simulink model "EB_12B_with_contracts"  (R2017b)
settings: Solver=ode3  StartTime=0.0  StopTime=0  FixedStep=.01  RelTol=1e-3  EnableMultiTasking=on
model workspace (MAT data in the model file):
  ContractValidatorBlocksMap = containers.Map
  ContractValidatorBlocksMap.serialization.keys = {'EB_12B_with_contracts/EB_12B_EBSpec/validator'}
  ContractValidatorBlocksMap.serialization.values{1}.block = 'EB_12B_with_contracts/EB_12B_EBSpec/validator'
  ContractValidatorBlocksMap.serialization.values{1}.assumePorts = 0
  ContractValidatorBlocksMap.serialization.values{1}.guaranteePorts = 3
  ContractValidatorBlocksMap.serialization.values{1}.modeBlocksPorts = 0
  ContractValidatorBlocksMap.serialization.values{1}.portHandles.Inport = [3286.00024414 3289.00024414 3293.00024414]
  ContractValidatorBlocksMap.serialization.values{1}.portHandles.Outport = 3586.00024414
  ContractValidatorBlocksMap.serialization.values{1}.portHandles.Enable = []
  ContractValidatorBlocksMap.serialization.values{1}.portHandles.Trigger = []
  ContractValidatorBlocksMap.serialization.values{1}.portHandles.State = []
  ContractValidatorBlocksMap.serialization.values{1}.portHandles.LConn = []
  ContractValidatorBlocksMap.serialization.values{1}.portHandles.RConn = []
  ContractValidatorBlocksMap.serialization.values{1}.portHandles.Ifaction = []
  ContractValidatorBlocksMap.serialization.values{1}.portHandles.Reset = []
  ContractValidatorBlocksMap.serialization.values{1}.portConnectivity(1).Type = '1'
  ContractValidatorBlocksMap.serialization.values{1}.portConnectivity(1).Position = [1955 -95]
  ContractValidatorBlocksMap.serialization.values{1}.portConnectivity(1).SrcBlock = 2019.00036621
  ContractValidatorBlocksMap.serialization.values{1}.portConnectivity(1).SrcPort = 0
  ContractValidatorBlocksMap.serialization.values{1}.portConnectivity(1).DstBlock = []
  ContractValidatorBlocksMap.serialization.values{1}.portConnectivity(1).DstPort = []
  ContractValidatorBlocksMap.serialization.values{1}.portConnectivity(2).Type = '2'
  ContractValidatorBlocksMap.serialization.values{1}.portConnectivity(2).Position = [1955 75]
  ContractValidatorBlocksMap.serialization.values{1}.portConnectivity(2).SrcBlock = 2023.00036621
  ContractValidatorBlocksMap.serialization.values{1}.portConnectivity(2).SrcPort = 0
  ContractValidatorBlocksMap.serialization.values{1}.portConnectivity(2).DstBlock = []
  ContractValidatorBlocksMap.serialization.values{1}.portConnectivity(2).DstPort = []
  ContractValidatorBlocksMap.serialization.values{1}.portConnectivity(3).Type = '3'
  ContractValidatorBlocksMap.serialization.values{1}.portConnectivity(3).Position = [1955 245]
  ContractValidatorBlocksMap.serialization.values{1}.portConnectivity(3).SrcBlock = 2031.00036621
  ContractValidatorBlocksMap.serialization.values{1}.portConnectivity(3).SrcPort = 0
  ContractValidatorBlocksMap.serialization.values{1}.portConnectivity(3).DstBlock = []
  ContractValidatorBlocksMap.serialization.values{1}.portConnectivity(3).DstPort = []
  ContractValidatorBlocksMap.serialization.values{1}.portConnectivity(4).Type = '1'
  ContractValidatorBlocksMap.serialization.values{1}.portConnectivity(4).Position = [2090 75]
  ContractValidatorBlocksMap.serialization.values{1}.portConnectivity(4).SrcBlock = []
  ContractValidatorBlocksMap.serialization.values{1}.portConnectivity(4).SrcPort = []
  ContractValidatorBlocksMap.serialization.values{1}.portConnectivity(4).DstBlock = 2226.00024414
  ContractValidatorBlocksMap.serialization.values{1}.portConnectivity(4).DstPort = 0
  ContractValidatorBlocksMap.serialization.uniformity = 0
  ContractValidatorBlocksMap.serialization.keyType = 'char'
  ContractValidatorBlocksMap.serialization.valueType = 'any'
undefined symbols (not defined in the file): contractAfterSimulation, contractBeforeSimulation, ContractBlock, ContractGuaranteeBlock, ContractValidatorBlock, d, I, I0, saveValidatorParameters, up, Wp
libraries: cocosimLibs x2
settings Model: Creator=elliocm  LastModifiedBy=hbourbou
settings DataIOCC: LimitDataPoints=on  SaveFormat=StructureWithTime  SignalLoggingSaveFormat=ModelDataLogs
settings OptimizationCC: LifeSpan=inf
settings DebuggingCC: UnderspecifiedInitializationDetection=Classic  MergeDetectMultiDrivingBlocksExec=none  SolverPrmCheckMsg=warning  MultiTaskDSMMsg=warning  MultiTaskCondExecSysMsg=none  SFUnexpectedBacktrackingDiag=warning  SFNoUnconditionalDefaultTransitionDiag=warning  SFExecutionAtInitializationDiag=none
settings HardwareCC: ProdBitPerPointer=32  ProdBitPerSizeT=32  ProdBitPerPtrDiffT=32  ProdLargestAtomicFloat=None  ProdIntDivRoundTo=Undefined  ProdEndianess=Unspecified  ProdWordSize=32  ProdHWDeviceType=32-bit Generic
settings ModelReferenceCC: PropagateSignalLabelsOutOfModel=off
settings CodeAppCC: StateflowObjectComments=on
settings GRTTargetCC: TargetLangStandard=C89/C90 (ANSI)  GeneratePreprocessorConditionals=Disable all
settings ConfigComp: CovMetricSettings=dw  CovHtmlReporting=on  CovSaveCumulativeToWorkspaceVar=on  CovSaveSingleToWorkspaceVar=on  CovExternalEMLEnable=off  DVMode=PropertyProving  DVTestSuiteOptimization=CombinedObjectives (Nonlinear Extended)

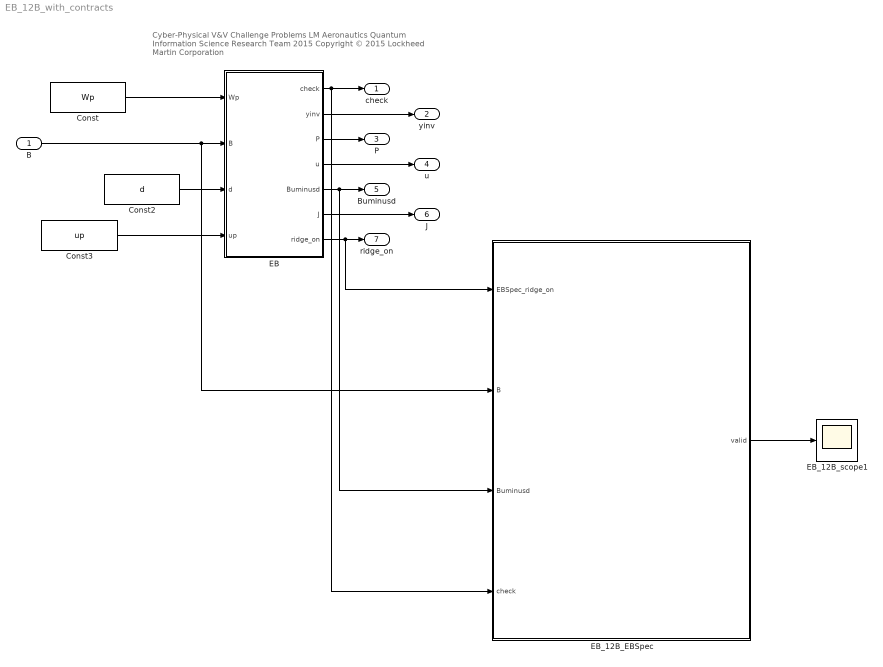
== system EB_12B_with_contracts ==
  note: Cyber-Physical V&V Challenge Problems
      | LM Aeronautics Quantum Information Science Research Team 2015
      | Copyright © 2015 Lockheed Martin Corporation
  B : Inport  OutDataTypeStr=double  PortDimensions=[3 5]
  Const : Constant  Value=Wp
  Const2 : Constant  Value=d
  Const3 : Constant  Value=up
  EB : Subsystem
  EB_12B_EBSpec : Subsystem  mask(ContractBlock){ContractBlockType=ContractBlock}
      mask init:
      | set_param(gcb, 'LinkStatus', 'none');
      mask DialogControl DescTextVar Prompt: Contract block
      mask Display:
      | text(0.5, 0.5, '{\bf\fontsize{20}Contract}', 'hor', 'center', 'texmode','on');
      | blocks = find_system(gcb, 'LookUnderMasks','all', 'SearchDepth',1,'BlockType','Inport');
      | for i = 1 : length(blocks)
      |     blockName = get_param(blocks(i), 'Name');
      |     [path, blockName] = fileparts(char(blockName));
      |     port_label('input', i, blockName);
      | end
      | 
      | blocks = find_system(gcb, 'LookUnderMasks','all', 'SearchDepth',1,'BlockType','Outport');
      | for i = 1 : length(blocks)
      |     blockName = get_param(blocks(i), 'Name');
      |     [path, blockName] = fileparts(char(blockName));
      |     port_label('output', i, blockName);
      | end
  EB_12B_scope1 : Scope
  check : Outport  VectorParamsAs1DForOutWhenUnconnected=off
  yinv : Outport  Port=2  VectorParamsAs1DForOutWhenUnconnected=off
  P : Outport  Port=3  VectorParamsAs1DForOutWhenUnconnected=off
  u : Outport  Port=4  VectorParamsAs1DForOutWhenUnconnected=off
  Buminusd : Outport  Port=5  VectorParamsAs1DForOutWhenUnconnected=off
  J : Outport  Port=6  VectorParamsAs1DForOutWhenUnconnected=off
  ridge_on : Outport  Port=7  VectorParamsAs1DForOutWhenUnconnected=off
  wires:
  Const/1 -> EB/1(Wp)
  B/1 -> EB_12B_EBSpec/2(B), EB/2(B)
  EB/2(yinv) -> yinv/1
  EB/1(check) -> check/1, EB_12B_EBSpec/4(check)
  Const2/1 -> EB/3(d)
  EB/3(P) -> P/1
  EB/4(u) -> u/1
  Const3/1 -> EB/4(up)
  EB/5(Buminusd) -> EB_12B_EBSpec/3(Buminusd), Buminusd/1
  EB/6(J) -> J/1
  EB/7(ridge_on) -> EB_12B_EBSpec/1(EBSpec_ridge_on), ridge_on/1
  EB_12B_EBSpec/1(valid) -> EB_12B_scope1/1

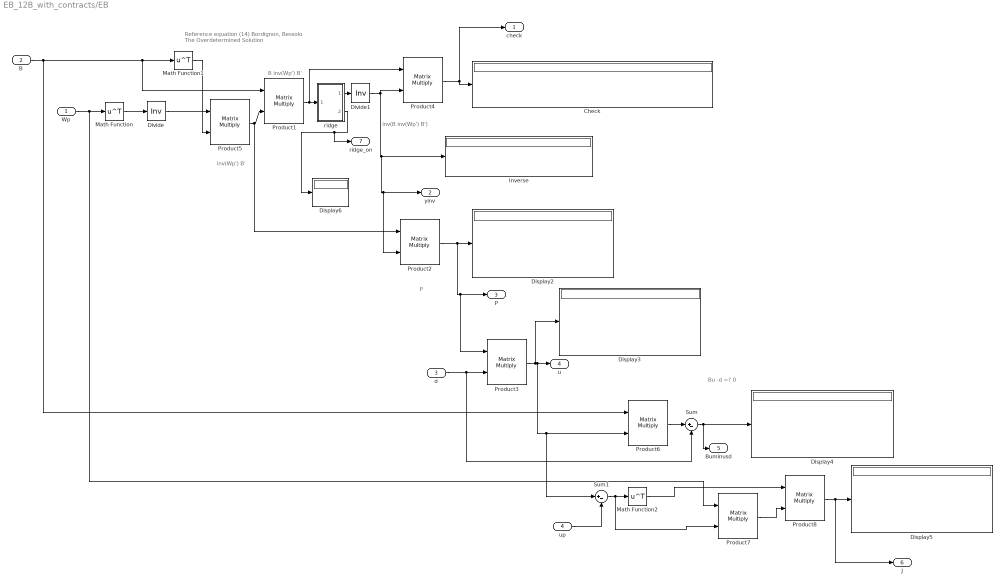
== system EB_12B_with_contracts/EB ==
  note: Reference equation (14) Bordignon, Bessolo
      | The Overdetermined Solution
  note: Bu -d =? 0
  note: P
  note: B inv(Wp') B'
  note: inv(B inv(Wp') B')
  note: inv(Wp') B'
  Wp : Inport
  B : Inport  Port=2
  d : Inport  Port=3
  up : Inport  Port=4
  Check : Display
      settings: Decimation=15
  Display{2..6} (5 alike) : Display
  Divide : Product  Inputs=/  Multiplication=Matrix(*)
  Divide1 : Product  Inputs=/  Multiplication=Matrix(*)
  Inverse : Display
  Math Function : Math  Operator=transpose  SaturateOnIntegerOverflow=on
  Math Function1 : Math  Operator=transpose  SaturateOnIntegerOverflow=on
  Math Function2 : Math  Operator=transpose  SaturateOnIntegerOverflow=on
  Product{1..8} (8 alike) : Product  Multiplication=Matrix(*)
  Sum : Sum  Inputs=|+-
  Sum1 : Sum  Inputs=|+-
  ridge : Subsystem
  check : Outport  VectorParamsAs1DForOutWhenUnconnected=off
  yinv : Outport  Port=2  VectorParamsAs1DForOutWhenUnconnected=off
  P : Outport  Port=3  VectorParamsAs1DForOutWhenUnconnected=off
  u : Outport  Port=4  VectorParamsAs1DForOutWhenUnconnected=off
  Buminusd : Outport  Port=5  VectorParamsAs1DForOutWhenUnconnected=off
  J : Outport  Port=6  VectorParamsAs1DForOutWhenUnconnected=off
  ridge_on : Outport  Port=7  VectorParamsAs1DForOutWhenUnconnected=off
  wires:
  Product1/1 -> Product4/1, ridge/1(In1)
  ridge/1(Out1) -> Divide1/1
  Divide/1 -> Product5/1
  Divide1/1 -> Product2/2, yinv/1, Inverse/1, Product4/2
  Math Function1/1 -> Product5/2
  B/1 -> Product6/1, Product1/1, Math Function1/1
  Math Function/1 -> Divide/1
  Wp/1 -> Product7/1, Math Function/1
  Product5/1 -> Product2/1, Product1/2
  Product4/1 -> check/1, Check/1
  Product2/1 -> Product3/1, P/1, Display2/1
  d/1 -> Sum/2, Product3/2
  Product3/1 -> Display3/1, Sum1/1, Product6/2, u/1
  Product6/1 -> Sum/1
  Sum/1 -> Buminusd/1, Display4/1
  up/1 -> Sum1/2
  Sum1/1 -> Product7/2, Math Function2/1
  Math Function2/1 -> Product8/1
  Product7/1 -> Product8/2
  Product8/1 -> J/1, Display5/1
  ridge/2(ridge_on) -> ridge_on/1, Display6/1

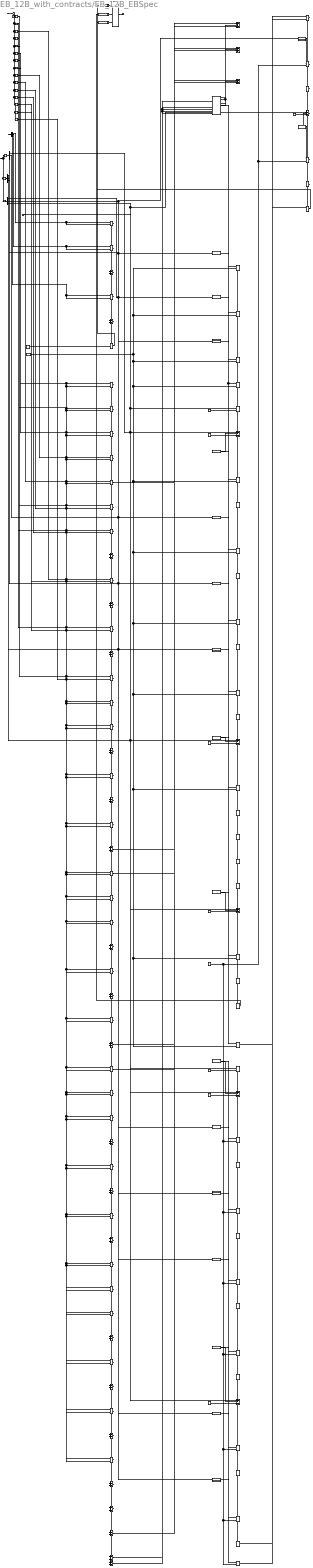
== system EB_12B_with_contracts/EB_12B_EBSpec ==
  EBSpec_ridge_on : Inport  OutDataTypeStr=boolean
  B : Inport  Port=2
  Buminusd : Inport  Port=3
  check : Inport  Port=4
  B_B_T_1_1_operator : Sum  OutDataTypeStr=double
  B_B_T_1_2_operator : Sum  OutDataTypeStr=double
  B_B_T_1_3_operator : Sum  OutDataTypeStr=double
  B_B_T_2_2_operator : Sum  OutDataTypeStr=double
  B_B_T_2_3_operator : Sum  OutDataTypeStr=double
  B_B_T_3_3_operator : Sum  OutDataTypeStr=double
  Buminusd_norm_operator : Sum  OutDataTypeStr=double
  Demux{,1..3} (4 alike) : Demux  Outputs=3
  EB001 : Subsystem  mask(ContractGuaranteeBlock){ContractBlockType=ContractGuaranteeBlock}
      mask init:
      | set_param(gcb, 'LinkStatus', 'none');
      mask DialogControl DescTextVar Prompt: Guarantee block
  EB002 : Subsystem  mask(ContractGuaranteeBlock){ContractBlockType=ContractGuaranteeBlock}
      mask init:
      | set_param(gcb, 'LinkStatus', 'none');
      mask DialogControl DescTextVar Prompt: Guarantee block
  EB004 : Subsystem  mask(ContractGuaranteeBlock){ContractBlockType=ContractGuaranteeBlock}
      mask init:
      | set_param(gcb, 'LinkStatus', 'none');
      mask DialogControl DescTextVar Prompt: Guarantee block
  Selector : Selector  NumberOfDimensions=2  InputPortWidth=3  IndexOptions=Index vector (dialog),Index vector (dialog)  Indices=1,1  OutputSizes=1,1
  Selector1 : Selector  NumberOfDimensions=2  InputPortWidth=3  IndexOptions=Index vector (dialog),Index vector (dialog)  Indices=1,2  OutputSizes=1,1
  Selector10 : Selector  NumberOfDimensions=2  InputPortWidth=3  IndexOptions=Index vector (dialog),Index vector (dialog)  Indices=3,1  OutputSizes=1,1
  Selector11 : Selector  NumberOfDimensions=2  InputPortWidth=3  IndexOptions=Index vector (dialog),Index vector (dialog)  Indices=3,2  OutputSizes=1,1
  Selector12 : Selector  NumberOfDimensions=2  InputPortWidth=3  IndexOptions=Index vector (dialog),Index vector (dialog)  Indices=3,3  OutputSizes=1,1
  Selector13 : Selector  NumberOfDimensions=2  InputPortWidth=3  IndexOptions=Index vector (dialog),Index vector (dialog)  Indices=3,4  OutputSizes=1,1
  Selector14 : Selector  NumberOfDimensions=2  InputPortWidth=3  IndexOptions=Index vector (dialog),Index vector (dialog)  Indices=3,5  OutputSizes=1,1
  Selector15 : Selector  NumberOfDimensions=2  InputPortWidth=3  IndexOptions=Index vector (dialog),Select all  Indices=1,1  OutputSizes=1,1
  Selector16 : Selector  NumberOfDimensions=2  InputPortWidth=3  IndexOptions=Index vector (dialog),Select all  Indices=2,1  OutputSizes=1,1
  Selector17 : Selector  NumberOfDimensions=2  InputPortWidth=3  IndexOptions=Index vector (dialog),Select all  Indices=3,1  OutputSizes=1,1
  Selector2 : Selector  NumberOfDimensions=2  InputPortWidth=3  IndexOptions=Index vector (dialog),Index vector (dialog)  Indices=1,3  OutputSizes=1,1
  Selector3 : Selector  NumberOfDimensions=2  InputPortWidth=3  IndexOptions=Index vector (dialog),Index vector (dialog)  Indices=1,4  OutputSizes=1,1
  Selector4 : Selector  NumberOfDimensions=2  InputPortWidth=3  IndexOptions=Index vector (dialog),Index vector (dialog)  Indices=1,5  OutputSizes=1,1
  Selector5 : Selector  NumberOfDimensions=2  InputPortWidth=3  IndexOptions=Index vector (dialog),Index vector (dialog)  Indices=2,1  OutputSizes=1,1
  Selector6 : Selector  NumberOfDimensions=2  InputPortWidth=3  IndexOptions=Index vector (dialog),Index vector (dialog)  Indices=2,2  OutputSizes=1,1
  Selector7 : Selector  NumberOfDimensions=2  InputPortWidth=3  IndexOptions=Index vector (dialog),Index vector (dialog)  Indices=2,3  OutputSizes=1,1
  Selector8 : Selector  NumberOfDimensions=2  InputPortWidth=3  IndexOptions=Index vector (dialog),Index vector (dialog)  Indices=2,4  OutputSizes=1,1
  Selector9 : Selector  NumberOfDimensions=2  InputPortWidth=3  IndexOptions=Index vector (dialog),Index vector (dialog)  Indices=2,5  OutputSizes=1,1
  abs_call : Subsystem
  abs_call1 : Subsystem
  abs_call11 : Subsystem
  abs_call111 : Subsystem
  abs_call1111 : Subsystem
  abs_call11111 : Subsystem
  abs_call111111 : Subsystem
  abs_call1111111 : Subsystem
  abs_call11111111 : Subsystem
  abs_call111111111 : Subsystem
  abs_call1111111111 : Subsystem
  abs_call11111111111 : Subsystem
  abs_call111111111111 : Subsystem
  abs_call1111111111111 : Subsystem
  abs_call11111111111111 : Subsystem
  abs_call111111111111111 : Subsystem
  abs_call1111111111111111 : Subsystem
  abs_call11111111111111111 : Subsystem
  det_3x3_call : Subsystem
  spec446_operator : cocosimLibs/Implies  SystemSampleTime=-1  Latency=0  AutoFrameSizeCalculation=off
  spec529_operator : cocosimLibs/Implies  SystemSampleTime=-1  Latency=0  AutoFrameSizeCalculation=off
  spec534_operator : RelationalOperator  Operator=<  OutDataTypeStr=boolean  RndMeth=Simplest
  spec534_rhs_2 : Constant  Value=0.0001  OutDataTypeStr=double
  validator : M-S-Function  LoadFcn=saveValidatorParameters(gcb);  InitFcn=contractBeforeSimulation();  StopFcn=contractAfterSimulation();  FunctionName=contract  mask(ContractValidatorBlock){assumePorts=0, guaranteePorts=3, modePorts=0, ContractBlockType=ContractValidatorBlock, createInportsCheckbox=off}
      mask prompts: assumePorts "Assume ports     :"; guaranteePorts "Guarantee ports :"; modePorts "Mode ports        :"; createInportsCheckbox "Create inports and connect them automatically"
      mask init:
      | set_param(gcb,'LinkStatus','none');
      | contract_callback('inputs_callback',gcb);
      mask DialogControl DescTextVar Prompt: The validator block implements the following logic: <br> <br> <b>Sofar</b>(assume<sub>1</sub> <b>&#8743;</b> assume<sub>2</sub> <b>&#8743;</b> ... assume<sub>k</sub>) <b>&rarr;</b> (guarantee<sub>1</sub> <b>&#8743;</b> guarantee<sub>2</sub> <b>&#8743;</b> ... guarantee<sub>m</sub> <b>&#8743;</b>  mode<sub>1</sub> <b>&#8743;</b> mode<sub>2</sub> <b>&#8743;</b> ... <b>&#8743;</b> mode<sub>n</sub> )<br> where mode<sub>i</sub> = require<sub>i</sub> <b>&rarr;</b> ensure<sub>i</sub>
      mask Display:
      | color('black');
      | port_label('input',1,'guarantee');
      | port_label('input',2,'guarantee');
      | port_label('input',3,'guarantee');
      | port_label('output',1,'valid');
  xxEBSpec_100_operator : Sum  OutDataTypeStr=double
  xxEBSpec_101_operator : Sum  OutDataTypeStr=double
  xxEBSpec_102_operator : Sum  OutDataTypeStr=double
  xxEBSpec_103_operator : Product  OutDataTypeStr=double
  xxEBSpec_104_operator : Product  OutDataTypeStr=double
  xxEBSpec_105_operator : Product  OutDataTypeStr=double
  xxEBSpec_106_operator : Product  OutDataTypeStr=double
  xxEBSpec_107_operator : Product  OutDataTypeStr=double
  xxEBSpec_108_operator : Sum  OutDataTypeStr=double
  xxEBSpec_109_operator : Sum  OutDataTypeStr=double
  xxEBSpec_10_operator : Sum  Inputs=+-  OutDataTypeStr=double
  xxEBSpec_10_rhs_2 : Constant  Value=1.0  OutDataTypeStr=double
  xxEBSpec_110_operator : Sum  OutDataTypeStr=double
  xxEBSpec_111_operator : Product  OutDataTypeStr=double
  xxEBSpec_112_operator : Product  OutDataTypeStr=double
  xxEBSpec_113_operator : Product  OutDataTypeStr=double
  xxEBSpec_114_operator : Product  OutDataTypeStr=double
  xxEBSpec_115_operator : Product  OutDataTypeStr=double
  xxEBSpec_116_operator : Sum  OutDataTypeStr=double
  xxEBSpec_117_operator : Sum  OutDataTypeStr=double
  xxEBSpec_118_operator : Sum  OutDataTypeStr=double
  xxEBSpec_12_operator : RelationalOperator  Operator=<  OutDataTypeStr=boolean  RndMeth=Simplest
  xxEBSpec_14_operator : RelationalOperator  Operator=<  OutDataTypeStr=boolean  RndMeth=Simplest
  xxEBSpec_16_operator : RelationalOperator  Operator=<  OutDataTypeStr=boolean  RndMeth=Simplest
  xxEBSpec_18_operator : RelationalOperator  Operator=<  OutDataTypeStr=boolean  RndMeth=Simplest
  xxEBSpec_19_operator : Sum  Inputs=+-  OutDataTypeStr=double
  xxEBSpec_19_rhs_2 : Constant  Value=1.0  OutDataTypeStr=double
  xxEBSpec_1_operator : Sum  Inputs=+-  OutDataTypeStr=double
  xxEBSpec_1_rhs_2 : Constant  Value=1.0  OutDataTypeStr=double
  xxEBSpec_21_operator : RelationalOperator  Operator=<  OutDataTypeStr=boolean  RndMeth=Simplest
  xxEBSpec_22_operator : RelationalOperator  Operator===  OutDataTypeStr=boolean  RndMeth=Simplest
  xxEBSpec_22_rhs_2 : Constant  Value=true  OutDataTypeStr=boolean
  xxEBSpec_23_operator : Logic  AllPortsSameDT=off  OutDataTypeStr=boolean
  xxEBSpec_24_operator : Logic  AllPortsSameDT=off  OutDataTypeStr=boolean
  xxEBSpec_25_operator : Logic  AllPortsSameDT=off  OutDataTypeStr=boolean
  xxEBSpec_26_operator : Logic  AllPortsSameDT=off  OutDataTypeStr=boolean
  xxEBSpec_27_operator : Logic  AllPortsSameDT=off  OutDataTypeStr=boolean
  xxEBSpec_28_operator : Logic  AllPortsSameDT=off  OutDataTypeStr=boolean
  xxEBSpec_29_operator : Logic  AllPortsSameDT=off  OutDataTypeStr=boolean
  xxEBSpec_30_operator : Logic  AllPortsSameDT=off  OutDataTypeStr=boolean
  xxEBSpec_31_operator : Logic  AllPortsSameDT=off  OutDataTypeStr=boolean
  xxEBSpec_32_operator : RelationalOperator  Operator=<=  OutDataTypeStr=boolean  RndMeth=Simplest
  xxEBSpec_33_operator : Sum  Inputs=+-  OutDataTypeStr=double
  xxEBSpec_33_rhs_2 : Constant  Value=1.0  OutDataTypeStr=double
  xxEBSpec_35_operator : RelationalOperator  Operator=<  OutDataTypeStr=boolean  RndMeth=Simplest
  xxEBSpec_37_operator : RelationalOperator  Operator=<  OutDataTypeStr=boolean  RndMeth=Simplest
  xxEBSpec_39_operator : RelationalOperator  Operator=<  OutDataTypeStr=boolean  RndMeth=Simplest
  xxEBSpec_3_operator : RelationalOperator  Operator=<  OutDataTypeStr=boolean  RndMeth=Simplest
  xxEBSpec_41_operator : RelationalOperator  Operator=<  OutDataTypeStr=boolean  RndMeth=Simplest
  xxEBSpec_42_operator : Sum  Inputs=+-  OutDataTypeStr=double
  xxEBSpec_42_rhs_2 : Constant  Value=1.0  OutDataTypeStr=double
  xxEBSpec_44_operator : RelationalOperator  Operator=<  OutDataTypeStr=boolean  RndMeth=Simplest
  xxEBSpec_46_operator : RelationalOperator  Operator=<  OutDataTypeStr=boolean  RndMeth=Simplest
  xxEBSpec_48_operator : RelationalOperator  Operator=<  OutDataTypeStr=boolean  RndMeth=Simplest
  xxEBSpec_50_operator : RelationalOperator  Operator=<  OutDataTypeStr=boolean  RndMeth=Simplest
  xxEBSpec_51_operator : Sum  Inputs=+-  OutDataTypeStr=double
  xxEBSpec_51_rhs_2 : Constant  Value=1.0  OutDataTypeStr=double
  xxEBSpec_53_operator : RelationalOperator  Operator=<  OutDataTypeStr=boolean  RndMeth=Simplest
  xxEBSpec_54_operator : RelationalOperator  Operator===  OutDataTypeStr=boolean  RndMeth=Simplest
  xxEBSpec_54_rhs_2 : Constant  Value=true  OutDataTypeStr=boolean
  xxEBSpec_55_operator : Logic  AllPortsSameDT=off  OutDataTypeStr=boolean
  xxEBSpec_56_operator : Logic  AllPortsSameDT=off  OutDataTypeStr=boolean
  xxEBSpec_57_operator : Logic  AllPortsSameDT=off  OutDataTypeStr=boolean
  xxEBSpec_58_operator : Logic  AllPortsSameDT=off  OutDataTypeStr=boolean
  xxEBSpec_59_operator : Logic  AllPortsSameDT=off  OutDataTypeStr=boolean
  xxEBSpec_5_operator : RelationalOperator  Operator=<  OutDataTypeStr=boolean  RndMeth=Simplest
  xxEBSpec_60_operator : Logic  AllPortsSameDT=off  OutDataTypeStr=boolean
  xxEBSpec_61_operator : Logic  AllPortsSameDT=off  OutDataTypeStr=boolean
  xxEBSpec_62_operator : Logic  AllPortsSameDT=off  OutDataTypeStr=boolean
  xxEBSpec_63_operator : Logic  AllPortsSameDT=off  OutDataTypeStr=boolean
  xxEBSpec_64_operator : RelationalOperator  Operator=<=  OutDataTypeStr=boolean  RndMeth=Simplest
  xxEBSpec_65_operator : Product  OutDataTypeStr=double
  xxEBSpec_66_operator : Product  OutDataTypeStr=double
  xxEBSpec_67_operator : Product  OutDataTypeStr=double
  xxEBSpec_68_operator : Sum  OutDataTypeStr=double
  xxEBSpec_69_rhs : Constant  Value=0.000000000001  OutDataTypeStr=double
  xxEBSpec_70_rhs : Constant  Value=0.000001  OutDataTypeStr=double
  xxEBSpec_71_operator : Product  OutDataTypeStr=double
  xxEBSpec_72_operator : Product  OutDataTypeStr=double
  xxEBSpec_73_operator : Product  OutDataTypeStr=double
  xxEBSpec_74_operator : Product  OutDataTypeStr=double
  xxEBSpec_75_operator : Product  OutDataTypeStr=double
  xxEBSpec_76_operator : Sum  OutDataTypeStr=double
  xxEBSpec_77_operator : Sum  OutDataTypeStr=double
  xxEBSpec_78_operator : Sum  OutDataTypeStr=double
  xxEBSpec_79_operator : Product  OutDataTypeStr=double
  xxEBSpec_7_operator : RelationalOperator  Operator=<  OutDataTypeStr=boolean  RndMeth=Simplest
  xxEBSpec_80_operator : Product  OutDataTypeStr=double
  xxEBSpec_81_operator : Product  OutDataTypeStr=double
  xxEBSpec_82_operator : Product  OutDataTypeStr=double
  xxEBSpec_83_operator : Product  OutDataTypeStr=double
  xxEBSpec_84_operator : Sum  OutDataTypeStr=double
  xxEBSpec_85_operator : Sum  OutDataTypeStr=double
  xxEBSpec_86_operator : Sum  OutDataTypeStr=double
  xxEBSpec_87_operator : Product  OutDataTypeStr=double
  xxEBSpec_88_operator : Product  OutDataTypeStr=double
  xxEBSpec_89_operator : Product  OutDataTypeStr=double
  xxEBSpec_90_operator : Product  OutDataTypeStr=double
  xxEBSpec_91_operator : Product  OutDataTypeStr=double
  xxEBSpec_92_operator : Sum  OutDataTypeStr=double
  xxEBSpec_93_operator : Sum  OutDataTypeStr=double
  xxEBSpec_94_operator : Sum  OutDataTypeStr=double
  xxEBSpec_95_operator : Product  OutDataTypeStr=double
  xxEBSpec_96_operator : Product  OutDataTypeStr=double
  xxEBSpec_97_operator : Product  OutDataTypeStr=double
  xxEBSpec_98_operator : Product  OutDataTypeStr=double
  xxEBSpec_99_operator : Product  OutDataTypeStr=double
  xxEBSpec_9_operator : RelationalOperator  Operator=<  OutDataTypeStr=boolean  RndMeth=Simplest
  valid : Outport
  wires:
  validator/1 -> valid/1
  abs_call/1(abs_y) -> xxEBSpec_9_operator/1
  xxEBSpec_88_operator/1 -> xxEBSpec_94_operator/2
  xxEBSpec_93_operator/1 -> xxEBSpec_94_operator/1
  xxEBSpec_89_operator/1 -> xxEBSpec_93_operator/2
  xxEBSpec_92_operator/1 -> xxEBSpec_93_operator/1
  xxEBSpec_90_operator/1 -> xxEBSpec_92_operator/2
  xxEBSpec_91_operator/1 -> xxEBSpec_92_operator/1
  xxEBSpec_80_operator/1 -> xxEBSpec_86_operator/2
  xxEBSpec_85_operator/1 -> xxEBSpec_86_operator/1
  xxEBSpec_81_operator/1 -> xxEBSpec_85_operator/2
  xxEBSpec_84_operator/1 -> xxEBSpec_85_operator/1
  xxEBSpec_82_operator/1 -> xxEBSpec_84_operator/2
  xxEBSpec_83_operator/1 -> xxEBSpec_84_operator/1
  abs_call1/1(abs_y) -> xxEBSpec_7_operator/1
  xxEBSpec_72_operator/1 -> xxEBSpec_78_operator/2
  xxEBSpec_77_operator/1 -> xxEBSpec_78_operator/1
  xxEBSpec_73_operator/1 -> xxEBSpec_77_operator/2
  xxEBSpec_76_operator/1 -> xxEBSpec_77_operator/1
  xxEBSpec_74_operator/1 -> xxEBSpec_76_operator/2
  xxEBSpec_75_operator/1 -> xxEBSpec_76_operator/1
  xxEBSpec_66_operator/1 -> xxEBSpec_68_operator/2
  xxEBSpec_67_operator/1 -> xxEBSpec_68_operator/1
  xxEBSpec_35_operator/1 -> xxEBSpec_63_operator/2
  xxEBSpec_62_operator/1 -> xxEBSpec_63_operator/1
  xxEBSpec_37_operator/1 -> xxEBSpec_62_operator/2
  xxEBSpec_61_operator/1 -> xxEBSpec_62_operator/1
  xxEBSpec_39_operator/1 -> xxEBSpec_61_operator/2
  xxEBSpec_60_operator/1 -> xxEBSpec_61_operator/1
  xxEBSpec_41_operator/1 -> xxEBSpec_60_operator/2
  xxEBSpec_59_operator/1 -> xxEBSpec_60_operator/1
  abs_call11/1(abs_y) -> xxEBSpec_5_operator/1
  xxEBSpec_44_operator/1 -> xxEBSpec_59_operator/2
  xxEBSpec_58_operator/1 -> xxEBSpec_59_operator/1
  xxEBSpec_46_operator/1 -> xxEBSpec_58_operator/2
  xxEBSpec_57_operator/1 -> xxEBSpec_58_operator/1
  xxEBSpec_48_operator/1 -> xxEBSpec_57_operator/2
  xxEBSpec_56_operator/1 -> xxEBSpec_57_operator/1
  xxEBSpec_50_operator/1 -> xxEBSpec_56_operator/2
  xxEBSpec_55_operator/1 -> xxEBSpec_56_operator/1
  xxEBSpec_53_operator/1 -> xxEBSpec_55_operator/2
  xxEBSpec_54_operator/1 -> xxEBSpec_55_operator/1
  xxEBSpec_54_rhs_2/1 -> xxEBSpec_54_operator/2
  abs_call111111111/1(abs_y) -> xxEBSpec_53_operator/1
  xxEBSpec_51_rhs_2/1 -> xxEBSpec_51_operator/2
  abs_call1111111111/1(abs_y) -> xxEBSpec_50_operator/1
  abs_call11111111111/1(abs_y) -> xxEBSpec_48_operator/1
  abs_call111111111111/1(abs_y) -> xxEBSpec_46_operator/1
  abs_call1111111111111/1(abs_y) -> xxEBSpec_44_operator/1
  xxEBSpec_42_rhs_2/1 -> xxEBSpec_42_operator/2
  abs_call11111111111111/1(abs_y) -> xxEBSpec_41_operator/1
  abs_call11111111/1(abs_y) -> xxEBSpec_3_operator/1
  abs_call111111111111111/1(abs_y) -> xxEBSpec_39_operator/1
  abs_call1111111111111111/1(abs_y) -> xxEBSpec_37_operator/1
  abs_call11111111111111111/1(abs_y) -> xxEBSpec_35_operator/1
  xxEBSpec_33_rhs_2/1 -> xxEBSpec_33_operator/2
  xxEBSpec_3_operator/1 -> xxEBSpec_31_operator/2
  xxEBSpec_30_operator/1 -> xxEBSpec_31_operator/1
  xxEBSpec_5_operator/1 -> xxEBSpec_30_operator/2
  xxEBSpec_29_operator/1 -> xxEBSpec_30_operator/1
  xxEBSpec_7_operator/1 -> xxEBSpec_29_operator/2
  xxEBSpec_28_operator/1 -> xxEBSpec_29_operator/1
  xxEBSpec_9_operator/1 -> xxEBSpec_28_operator/2
  xxEBSpec_27_operator/1 -> xxEBSpec_28_operator/1
  xxEBSpec_12_operator/1 -> xxEBSpec_27_operator/2
  xxEBSpec_26_operator/1 -> xxEBSpec_27_operator/1
  xxEBSpec_14_operator/1 -> xxEBSpec_26_operator/2
  xxEBSpec_25_operator/1 -> xxEBSpec_26_operator/1
  xxEBSpec_16_operator/1 -> xxEBSpec_25_operator/2
  xxEBSpec_24_operator/1 -> xxEBSpec_25_operator/1
  xxEBSpec_18_operator/1 -> xxEBSpec_24_operator/2
  xxEBSpec_23_operator/1 -> xxEBSpec_24_operator/1
  xxEBSpec_21_operator/1 -> xxEBSpec_23_operator/2
  xxEBSpec_22_operator/1 -> xxEBSpec_23_operator/1
  xxEBSpec_22_rhs_2/1 -> xxEBSpec_22_operator/2
  abs_call111/1(abs_y) -> xxEBSpec_21_operator/1
  xxEBSpec_1_rhs_2/1 -> xxEBSpec_1_operator/2
  xxEBSpec_19_rhs_2/1 -> xxEBSpec_19_operator/2
  abs_call1111/1(abs_y) -> xxEBSpec_18_operator/1
  abs_call11111/1(abs_y) -> xxEBSpec_16_operator/1
  abs_call111111/1(abs_y) -> xxEBSpec_14_operator/1
  abs_call1111111/1(abs_y) -> xxEBSpec_12_operator/1
  xxEBSpec_112_operator/1 -> xxEBSpec_118_operator/2
  xxEBSpec_117_operator/1 -> xxEBSpec_118_operator/1
  xxEBSpec_113_operator/1 -> xxEBSpec_117_operator/2
  xxEBSpec_116_operator/1 -> xxEBSpec_117_operator/1
  xxEBSpec_114_operator/1 -> xxEBSpec_116_operator/2
  xxEBSpec_115_operator/1 -> xxEBSpec_116_operator/1
  xxEBSpec_104_operator/1 -> xxEBSpec_110_operator/2
  xxEBSpec_109_operator/1 -> xxEBSpec_110_operator/1
  xxEBSpec_10_rhs_2/1 -> xxEBSpec_10_operator/2
  xxEBSpec_105_operator/1 -> xxEBSpec_109_operator/2
  xxEBSpec_108_operator/1 -> xxEBSpec_109_operator/1
  xxEBSpec_106_operator/1 -> xxEBSpec_108_operator/2
  xxEBSpec_107_operator/1 -> xxEBSpec_108_operator/1
  xxEBSpec_96_operator/1 -> xxEBSpec_102_operator/2
  xxEBSpec_101_operator/1 -> xxEBSpec_102_operator/1
  xxEBSpec_97_operator/1 -> xxEBSpec_101_operator/2
  xxEBSpec_100_operator/1 -> xxEBSpec_101_operator/1
  xxEBSpec_98_operator/1 -> xxEBSpec_100_operator/2
  xxEBSpec_99_operator/1 -> xxEBSpec_100_operator/1
  EB004/1(guarantee) -> validator/3
  EB002/1(guarantee) -> validator/2
  EB001/1(guarantee) -> validator/1
  spec534_rhs_2/1 -> spec534_operator/2
  Buminusd_norm_operator/1 -> spec534_operator/1
  xxEBSpec_31_operator/1 -> spec529_operator/2
  xxEBSpec_32_operator/1 -> spec529_operator/1
  xxEBSpec_63_operator/1 -> spec446_operator/2
  xxEBSpec_64_operator/1 -> spec446_operator/1
  spec534_operator/1 -> EB004/1(In1)
  spec529_operator/1 -> EB002/1(In1)
  spec446_operator/1 -> EB001/1(In1)
  B_B_T_3_3_operator/1 -> det_3x3_call/9(det_3x3_a33)
  B_B_T_2_2_operator/1 -> det_3x3_call/5(det_3x3_a22)
  B_B_T_1_1_operator/1 -> det_3x3_call/1(det_3x3_a11)
  xxEBSpec_33_operator/1 -> abs_call11111111111111111/1(abs_x)
  xxEBSpec_42_operator/1 -> abs_call1111111111111/1(abs_x)
  xxEBSpec_51_operator/1 -> abs_call111111111/1(abs_x)
  xxEBSpec_1_operator/1 -> abs_call11111111/1(abs_x)
  xxEBSpec_10_operator/1 -> abs_call1111111/1(abs_x)
  xxEBSpec_19_operator/1 -> abs_call111/1(abs_x)
  xxEBSpec_65_operator/1 -> Buminusd_norm_operator/2
  xxEBSpec_68_operator/1 -> Buminusd_norm_operator/1
  xxEBSpec_111_operator/1 -> B_B_T_3_3_operator/2
  xxEBSpec_118_operator/1 -> B_B_T_3_3_operator/1
  xxEBSpec_103_operator/1 -> B_B_T_2_3_operator/2
  xxEBSpec_110_operator/1 -> B_B_T_2_3_operator/1
  xxEBSpec_95_operator/1 -> B_B_T_2_2_operator/2
  xxEBSpec_102_operator/1 -> B_B_T_2_2_operator/1
  xxEBSpec_87_operator/1 -> B_B_T_1_3_operator/2
  xxEBSpec_94_operator/1 -> B_B_T_1_3_operator/1
  xxEBSpec_79_operator/1 -> B_B_T_1_2_operator/2
  xxEBSpec_86_operator/1 -> B_B_T_1_2_operator/1
  xxEBSpec_71_operator/1 -> B_B_T_1_1_operator/2
  xxEBSpec_78_operator/1 -> B_B_T_1_1_operator/1
  xxEBSpec_70_rhs/1 -> xxEBSpec_41_operator/2, xxEBSpec_39_operator/2, xxEBSpec_44_operator/2, xxEBSpec_46_operator/2, xxEBSpec_48_operator/2, xxEBSpec_50_operator/2, xxEBSpec_53_operator/2, xxEBSpec_37_operator/2, xxEBSpec_35_operator/2
  Demux3/3 -> xxEBSpec_33_operator/1, xxEBSpec_1_operator/1
  xxEBSpec_69_rhs/1 -> xxEBSpec_64_operator/2, xxEBSpec_3_operator/2, xxEBSpec_12_operator/2, xxEBSpec_14_operator/2, xxEBSpec_16_operator/2, xxEBSpec_18_operator/2, xxEBSpec_21_operator/2, xxEBSpec_32_operator/2, xxEBSpec_5_operator/2, xxEBSpec_9_operator/2, xxEBSpec_7_operator/2
  Demux2/2 -> xxEBSpec_42_operator/1, xxEBSpec_10_operator/1
  Demux2/1 -> abs_call111111111111/1(abs_x), abs_call111111/1(abs_x)
  Demux1/3 -> abs_call11111111111/1(abs_x), abs_call11111/1(abs_x)
  Demux1/2 -> abs_call1111111111/1(abs_x), abs_call1111/1(abs_x)
  Demux1/1 -> xxEBSpec_51_operator/1, xxEBSpec_19_operator/1
  EBSpec_ridge_on/1 -> xxEBSpec_54_operator/1, xxEBSpec_22_operator/1
  det_3x3_call/1(det_3x3_det) -> xxEBSpec_64_operator/1, xxEBSpec_32_operator/1
  Demux3/2 -> abs_call1111111111111111/1(abs_x), abs_call11/1(abs_x)
  Demux3/1 -> abs_call111111111111111/1(abs_x), abs_call1/1(abs_x)
  Demux2/3 -> abs_call11111111111111/1(abs_x), abs_call/1(abs_x)
  B_B_T_1_2_operator/1 -> det_3x3_call/4(det_3x3_a12), det_3x3_call/2(det_3x3_a21)
  B_B_T_1_3_operator/1 -> det_3x3_call/7(det_3x3_a13), det_3x3_call/3(det_3x3_a31)
  B_B_T_2_3_operator/1 -> det_3x3_call/8(det_3x3_a23), det_3x3_call/6(det_3x3_a32)
  Selector14/1 -> xxEBSpec_111_operator/2, xxEBSpec_103_operator/2, xxEBSpec_111_operator/1, xxEBSpec_87_operator/2
  Selector9/1 -> xxEBSpec_79_operator/2, xxEBSpec_103_operator/1, xxEBSpec_95_operator/2, xxEBSpec_95_operator/1
  Selector13/1 -> xxEBSpec_112_operator/2, xxEBSpec_104_operator/2, xxEBSpec_112_operator/1, xxEBSpec_88_operator/2
  Selector8/1 -> xxEBSpec_80_operator/2, xxEBSpec_104_operator/1, xxEBSpec_96_operator/2, xxEBSpec_96_operator/1
  Selector12/1 -> xxEBSpec_113_operator/2, xxEBSpec_105_operator/2, xxEBSpec_113_operator/1, xxEBSpec_89_operator/2
  Selector7/1 -> xxEBSpec_81_operator/2, xxEBSpec_105_operator/1, xxEBSpec_97_operator/2, xxEBSpec_97_operator/1
  Selector11/1 -> xxEBSpec_114_operator/2, xxEBSpec_106_operator/2, xxEBSpec_114_operator/1, xxEBSpec_90_operator/2
  Selector6/1 -> xxEBSpec_82_operator/2, xxEBSpec_106_operator/1, xxEBSpec_98_operator/2, xxEBSpec_98_operator/1
  Selector10/1 -> xxEBSpec_115_operator/2, xxEBSpec_107_operator/2, xxEBSpec_115_operator/1, xxEBSpec_91_operator/2
  Selector5/1 -> xxEBSpec_83_operator/2, xxEBSpec_107_operator/1, xxEBSpec_99_operator/2, xxEBSpec_99_operator/1
  Selector4/1 -> xxEBSpec_71_operator/2, xxEBSpec_71_operator/1, xxEBSpec_79_operator/1, xxEBSpec_87_operator/1
  Selector3/1 -> xxEBSpec_72_operator/2, xxEBSpec_72_operator/1, xxEBSpec_80_operator/1, xxEBSpec_88_operator/1
  Selector2/1 -> xxEBSpec_73_operator/2, xxEBSpec_73_operator/1, xxEBSpec_81_operator/1, xxEBSpec_89_operator/1
  Selector1/1 -> xxEBSpec_74_operator/2, xxEBSpec_74_operator/1, xxEBSpec_82_operator/1, xxEBSpec_90_operator/1
  Selector/1 -> xxEBSpec_75_operator/2, xxEBSpec_75_operator/1, xxEBSpec_83_operator/1, xxEBSpec_91_operator/1
  Demux/3 -> xxEBSpec_65_operator/2, xxEBSpec_65_operator/1
  Demux/2 -> xxEBSpec_66_operator/2, xxEBSpec_66_operator/1
  Demux/1 -> xxEBSpec_67_operator/2, xxEBSpec_67_operator/1
  B/1 -> [B]
  [B] -> Selector14/1, Selector13/1, Selector12/1, Selector11/1, Selector10/1, Selector9/1, Selector8/1, Selector7/1, Selector6/1, Selector5/1, Selector4/1, Selector3/1, Selector2/1, Selector1/1, Selector/1
  Buminusd/1 -> Demux/1
  check/1 -> Selector17/1, Selector16/1, Selector15/1
  Selector15/1 -> Demux1/1
  Selector16/1 -> Demux2/1
  Selector17/1 -> Demux3/1

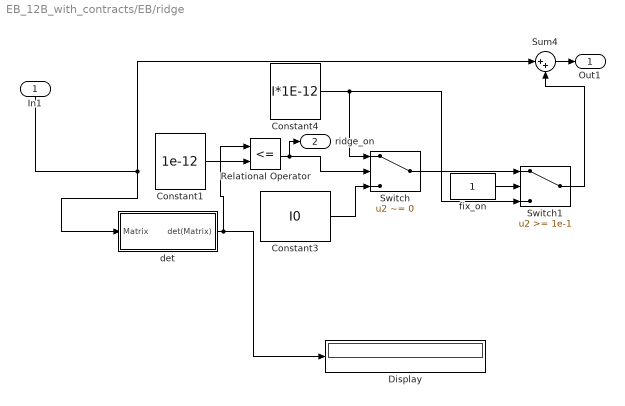
== system EB_12B_with_contracts/EB/ridge ==
  In1 : Inport
  Constant1 : Constant  Value=1e-12
  Constant3 : Constant  Value=I0
  Constant4 : Constant  Value=I*1E-12
  Display : Display
  Relational Operator : RelationalOperator  Operator=<=  OutDataTypeStr=boolean  RndMeth=Nearest
  Sum4 : Sum  Inputs=|++
  Switch : Switch  Criteria=u2 ~= 0  Threshold=1e-5
  Switch1 : Switch  Threshold=1e-1
  det : Subsystem
  fix_on : Constant
  Out1 : Outport  VectorParamsAs1DForOutWhenUnconnected=off
  ridge_on : Outport  Port=2  VectorParamsAs1DForOutWhenUnconnected=off
  wires:
  Sum4/1 -> Out1/1
  Constant4/1 -> Switch/1, Switch1/3
  In1/1 -> Sum4/1, det/1(Matrix)
  Switch1/1 -> Sum4/2
  Switch/1 -> Switch1/1
  fix_on/1 -> Switch1/2
  det/1(det(Matrix)) -> Relational Operator/1, Display/1
  Relational Operator/1 -> ridge_on/1, Switch/2
  Constant1/1 -> Relational Operator/2
  Constant3/1 -> Switch/3

== system EB_12B_with_contracts/EB_12B_EBSpec/EB001 ==
  In1 : Inport
  guarantee : Outport  OutDataTypeStr=boolean
  wires:
  In1/1 -> guarantee/1

== system EB_12B_with_contracts/EB_12B_EBSpec/EB002 ==
  In1 : Inport
  guarantee : Outport  OutDataTypeStr=boolean
  wires:
  In1/1 -> guarantee/1

== system EB_12B_with_contracts/EB_12B_EBSpec/EB004 ==
  In1 : Inport
  guarantee : Outport  OutDataTypeStr=boolean
  wires:
  In1/1 -> guarantee/1

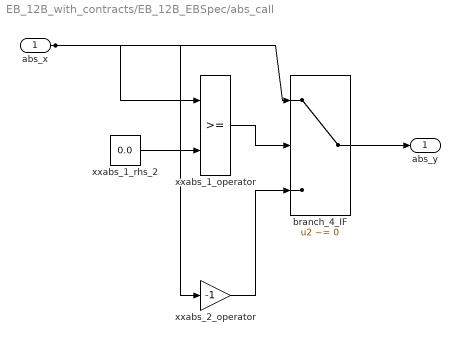
== system EB_12B_with_contracts/EB_12B_EBSpec/abs_call ==
  abs_x : Inport  OutDataTypeStr=double
  branch_4_IF : Switch  Criteria=u2 ~= 0
  xxabs_1_operator : RelationalOperator  OutDataTypeStr=boolean  RndMeth=Simplest
  xxabs_1_rhs_2 : Constant  Value=0.0  OutDataTypeStr=double
  xxabs_2_operator : Gain  Gain=-1  OutDataTypeStr=double
  abs_y : Outport
  wires:
  branch_4_IF/1 -> abs_y/1
  xxabs_1_rhs_2/1 -> xxabs_1_operator/2
  xxabs_2_operator/1 -> branch_4_IF/3
  xxabs_1_operator/1 -> branch_4_IF/2
  abs_x/1 -> xxabs_2_operator/1, xxabs_1_operator/1, branch_4_IF/1

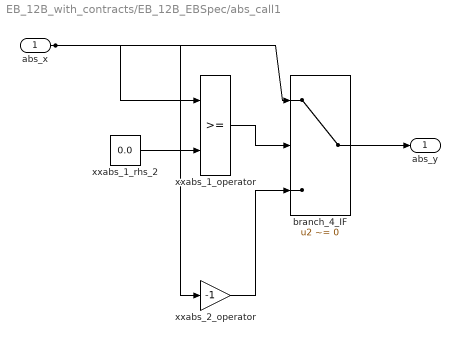
== system EB_12B_with_contracts/EB_12B_EBSpec/abs_call1 ==
  abs_x : Inport  OutDataTypeStr=double
  branch_4_IF : Switch  Criteria=u2 ~= 0
  xxabs_1_operator : RelationalOperator  OutDataTypeStr=boolean  RndMeth=Simplest
  xxabs_1_rhs_2 : Constant  Value=0.0  OutDataTypeStr=double
  xxabs_2_operator : Gain  Gain=-1  OutDataTypeStr=double
  abs_y : Outport
  wires:
  branch_4_IF/1 -> abs_y/1
  xxabs_1_rhs_2/1 -> xxabs_1_operator/2
  xxabs_2_operator/1 -> branch_4_IF/3
  xxabs_1_operator/1 -> branch_4_IF/2
  abs_x/1 -> xxabs_2_operator/1, xxabs_1_operator/1, branch_4_IF/1

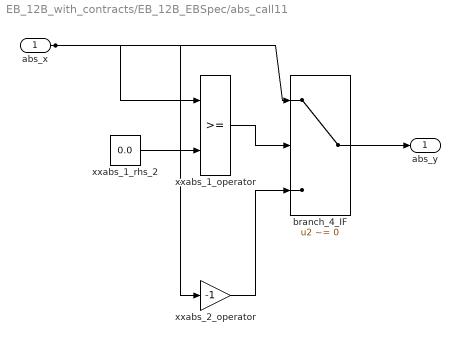
== system EB_12B_with_contracts/EB_12B_EBSpec/abs_call11 ==
  abs_x : Inport  OutDataTypeStr=double
  branch_4_IF : Switch  Criteria=u2 ~= 0
  xxabs_1_operator : RelationalOperator  OutDataTypeStr=boolean  RndMeth=Simplest
  xxabs_1_rhs_2 : Constant  Value=0.0  OutDataTypeStr=double
  xxabs_2_operator : Gain  Gain=-1  OutDataTypeStr=double
  abs_y : Outport
  wires:
  branch_4_IF/1 -> abs_y/1
  xxabs_1_rhs_2/1 -> xxabs_1_operator/2
  xxabs_2_operator/1 -> branch_4_IF/3
  xxabs_1_operator/1 -> branch_4_IF/2
  abs_x/1 -> xxabs_2_operator/1, xxabs_1_operator/1, branch_4_IF/1

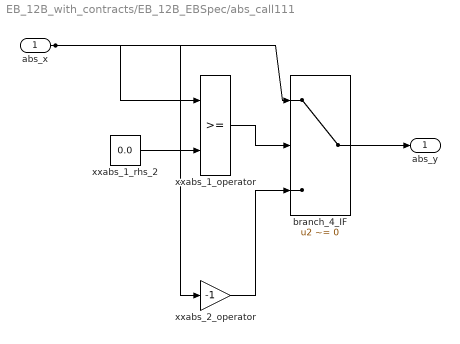
== system EB_12B_with_contracts/EB_12B_EBSpec/abs_call111 ==
  abs_x : Inport  OutDataTypeStr=double
  branch_4_IF : Switch  Criteria=u2 ~= 0
  xxabs_1_operator : RelationalOperator  OutDataTypeStr=boolean  RndMeth=Simplest
  xxabs_1_rhs_2 : Constant  Value=0.0  OutDataTypeStr=double
  xxabs_2_operator : Gain  Gain=-1  OutDataTypeStr=double
  abs_y : Outport
  wires:
  branch_4_IF/1 -> abs_y/1
  xxabs_1_rhs_2/1 -> xxabs_1_operator/2
  xxabs_2_operator/1 -> branch_4_IF/3
  xxabs_1_operator/1 -> branch_4_IF/2
  abs_x/1 -> xxabs_2_operator/1, xxabs_1_operator/1, branch_4_IF/1

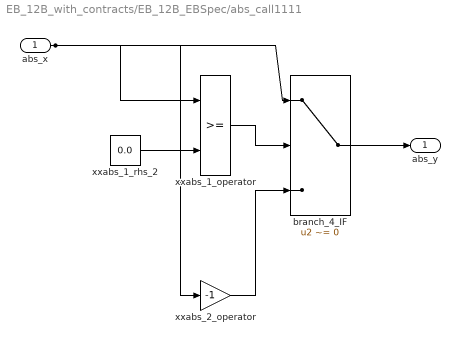
== system EB_12B_with_contracts/EB_12B_EBSpec/abs_call1111 ==
  abs_x : Inport  OutDataTypeStr=double
  branch_4_IF : Switch  Criteria=u2 ~= 0
  xxabs_1_operator : RelationalOperator  OutDataTypeStr=boolean  RndMeth=Simplest
  xxabs_1_rhs_2 : Constant  Value=0.0  OutDataTypeStr=double
  xxabs_2_operator : Gain  Gain=-1  OutDataTypeStr=double
  abs_y : Outport
  wires:
  branch_4_IF/1 -> abs_y/1
  xxabs_1_rhs_2/1 -> xxabs_1_operator/2
  xxabs_2_operator/1 -> branch_4_IF/3
  xxabs_1_operator/1 -> branch_4_IF/2
  abs_x/1 -> xxabs_2_operator/1, xxabs_1_operator/1, branch_4_IF/1

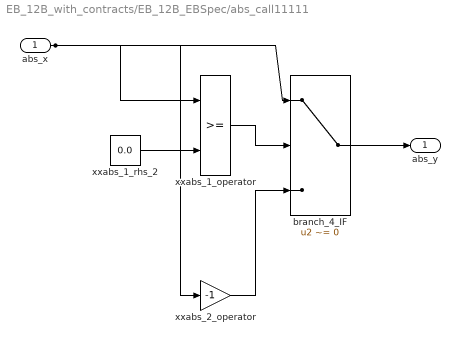
== system EB_12B_with_contracts/EB_12B_EBSpec/abs_call11111 ==
  abs_x : Inport  OutDataTypeStr=double
  branch_4_IF : Switch  Criteria=u2 ~= 0
  xxabs_1_operator : RelationalOperator  OutDataTypeStr=boolean  RndMeth=Simplest
  xxabs_1_rhs_2 : Constant  Value=0.0  OutDataTypeStr=double
  xxabs_2_operator : Gain  Gain=-1  OutDataTypeStr=double
  abs_y : Outport
  wires:
  branch_4_IF/1 -> abs_y/1
  xxabs_1_rhs_2/1 -> xxabs_1_operator/2
  xxabs_2_operator/1 -> branch_4_IF/3
  xxabs_1_operator/1 -> branch_4_IF/2
  abs_x/1 -> xxabs_2_operator/1, xxabs_1_operator/1, branch_4_IF/1

== system EB_12B_with_contracts/EB_12B_EBSpec/abs_call111111 ==
  abs_x : Inport  OutDataTypeStr=double
  branch_4_IF : Switch  Criteria=u2 ~= 0
  xxabs_1_operator : RelationalOperator  OutDataTypeStr=boolean  RndMeth=Simplest
  xxabs_1_rhs_2 : Constant  Value=0.0  OutDataTypeStr=double
  xxabs_2_operator : Gain  Gain=-1  OutDataTypeStr=double
  abs_y : Outport
  wires:
  branch_4_IF/1 -> abs_y/1
  xxabs_1_rhs_2/1 -> xxabs_1_operator/2
  xxabs_2_operator/1 -> branch_4_IF/3
  xxabs_1_operator/1 -> branch_4_IF/2
  abs_x/1 -> xxabs_2_operator/1, xxabs_1_operator/1, branch_4_IF/1

== system EB_12B_with_contracts/EB_12B_EBSpec/abs_call1111111 ==
  abs_x : Inport  OutDataTypeStr=double
  branch_4_IF : Switch  Criteria=u2 ~= 0
  xxabs_1_operator : RelationalOperator  OutDataTypeStr=boolean  RndMeth=Simplest
  xxabs_1_rhs_2 : Constant  Value=0.0  OutDataTypeStr=double
  xxabs_2_operator : Gain  Gain=-1  OutDataTypeStr=double
  abs_y : Outport
  wires:
  branch_4_IF/1 -> abs_y/1
  xxabs_1_rhs_2/1 -> xxabs_1_operator/2
  xxabs_2_operator/1 -> branch_4_IF/3
  xxabs_1_operator/1 -> branch_4_IF/2
  abs_x/1 -> xxabs_2_operator/1, xxabs_1_operator/1, branch_4_IF/1

== system EB_12B_with_contracts/EB_12B_EBSpec/abs_call11111111 ==
  abs_x : Inport  OutDataTypeStr=double
  branch_4_IF : Switch  Criteria=u2 ~= 0
  xxabs_1_operator : RelationalOperator  OutDataTypeStr=boolean  RndMeth=Simplest
  xxabs_1_rhs_2 : Constant  Value=0.0  OutDataTypeStr=double
  xxabs_2_operator : Gain  Gain=-1  OutDataTypeStr=double
  abs_y : Outport
  wires:
  branch_4_IF/1 -> abs_y/1
  xxabs_1_rhs_2/1 -> xxabs_1_operator/2
  xxabs_2_operator/1 -> branch_4_IF/3
  xxabs_1_operator/1 -> branch_4_IF/2
  abs_x/1 -> xxabs_2_operator/1, xxabs_1_operator/1, branch_4_IF/1

== system EB_12B_with_contracts/EB_12B_EBSpec/abs_call111111111 ==
  abs_x : Inport  OutDataTypeStr=double
  branch_4_IF : Switch  Criteria=u2 ~= 0
  xxabs_1_operator : RelationalOperator  OutDataTypeStr=boolean  RndMeth=Simplest
  xxabs_1_rhs_2 : Constant  Value=0.0  OutDataTypeStr=double
  xxabs_2_operator : Gain  Gain=-1  OutDataTypeStr=double
  abs_y : Outport
  wires:
  branch_4_IF/1 -> abs_y/1
  xxabs_1_rhs_2/1 -> xxabs_1_operator/2
  xxabs_2_operator/1 -> branch_4_IF/3
  xxabs_1_operator/1 -> branch_4_IF/2
  abs_x/1 -> xxabs_2_operator/1, xxabs_1_operator/1, branch_4_IF/1

== system EB_12B_with_contracts/EB_12B_EBSpec/abs_call1111111111 ==
  abs_x : Inport  OutDataTypeStr=double
  branch_4_IF : Switch  Criteria=u2 ~= 0
  xxabs_1_operator : RelationalOperator  OutDataTypeStr=boolean  RndMeth=Simplest
  xxabs_1_rhs_2 : Constant  Value=0.0  OutDataTypeStr=double
  xxabs_2_operator : Gain  Gain=-1  OutDataTypeStr=double
  abs_y : Outport
  wires:
  branch_4_IF/1 -> abs_y/1
  xxabs_1_rhs_2/1 -> xxabs_1_operator/2
  xxabs_2_operator/1 -> branch_4_IF/3
  xxabs_1_operator/1 -> branch_4_IF/2
  abs_x/1 -> xxabs_2_operator/1, xxabs_1_operator/1, branch_4_IF/1

== system EB_12B_with_contracts/EB_12B_EBSpec/abs_call11111111111 ==
  abs_x : Inport  OutDataTypeStr=double
  branch_4_IF : Switch  Criteria=u2 ~= 0
  xxabs_1_operator : RelationalOperator  OutDataTypeStr=boolean  RndMeth=Simplest
  xxabs_1_rhs_2 : Constant  Value=0.0  OutDataTypeStr=double
  xxabs_2_operator : Gain  Gain=-1  OutDataTypeStr=double
  abs_y : Outport
  wires:
  branch_4_IF/1 -> abs_y/1
  xxabs_1_rhs_2/1 -> xxabs_1_operator/2
  xxabs_2_operator/1 -> branch_4_IF/3
  xxabs_1_operator/1 -> branch_4_IF/2
  abs_x/1 -> xxabs_2_operator/1, xxabs_1_operator/1, branch_4_IF/1

== system EB_12B_with_contracts/EB_12B_EBSpec/abs_call111111111111 ==
  abs_x : Inport  OutDataTypeStr=double
  branch_4_IF : Switch  Criteria=u2 ~= 0
  xxabs_1_operator : RelationalOperator  OutDataTypeStr=boolean  RndMeth=Simplest
  xxabs_1_rhs_2 : Constant  Value=0.0  OutDataTypeStr=double
  xxabs_2_operator : Gain  Gain=-1  OutDataTypeStr=double
  abs_y : Outport
  wires:
  branch_4_IF/1 -> abs_y/1
  xxabs_1_rhs_2/1 -> xxabs_1_operator/2
  xxabs_2_operator/1 -> branch_4_IF/3
  xxabs_1_operator/1 -> branch_4_IF/2
  abs_x/1 -> xxabs_2_operator/1, xxabs_1_operator/1, branch_4_IF/1

== system EB_12B_with_contracts/EB_12B_EBSpec/abs_call1111111111111 ==
  abs_x : Inport  OutDataTypeStr=double
  branch_4_IF : Switch  Criteria=u2 ~= 0
  xxabs_1_operator : RelationalOperator  OutDataTypeStr=boolean  RndMeth=Simplest
  xxabs_1_rhs_2 : Constant  Value=0.0  OutDataTypeStr=double
  xxabs_2_operator : Gain  Gain=-1  OutDataTypeStr=double
  abs_y : Outport
  wires:
  branch_4_IF/1 -> abs_y/1
  xxabs_1_rhs_2/1 -> xxabs_1_operator/2
  xxabs_2_operator/1 -> branch_4_IF/3
  xxabs_1_operator/1 -> branch_4_IF/2
  abs_x/1 -> xxabs_2_operator/1, xxabs_1_operator/1, branch_4_IF/1

== system EB_12B_with_contracts/EB_12B_EBSpec/abs_call11111111111111 ==
  abs_x : Inport  OutDataTypeStr=double
  branch_4_IF : Switch  Criteria=u2 ~= 0
  xxabs_1_operator : RelationalOperator  OutDataTypeStr=boolean  RndMeth=Simplest
  xxabs_1_rhs_2 : Constant  Value=0.0  OutDataTypeStr=double
  xxabs_2_operator : Gain  Gain=-1  OutDataTypeStr=double
  abs_y : Outport
  wires:
  branch_4_IF/1 -> abs_y/1
  xxabs_1_rhs_2/1 -> xxabs_1_operator/2
  xxabs_2_operator/1 -> branch_4_IF/3
  xxabs_1_operator/1 -> branch_4_IF/2
  abs_x/1 -> xxabs_2_operator/1, xxabs_1_operator/1, branch_4_IF/1

== system EB_12B_with_contracts/EB_12B_EBSpec/abs_call111111111111111 ==
  abs_x : Inport  OutDataTypeStr=double
  branch_4_IF : Switch  Criteria=u2 ~= 0
  xxabs_1_operator : RelationalOperator  OutDataTypeStr=boolean  RndMeth=Simplest
  xxabs_1_rhs_2 : Constant  Value=0.0  OutDataTypeStr=double
  xxabs_2_operator : Gain  Gain=-1  OutDataTypeStr=double
  abs_y : Outport
  wires:
  branch_4_IF/1 -> abs_y/1
  xxabs_1_rhs_2/1 -> xxabs_1_operator/2
  xxabs_2_operator/1 -> branch_4_IF/3
  xxabs_1_operator/1 -> branch_4_IF/2
  abs_x/1 -> xxabs_2_operator/1, xxabs_1_operator/1, branch_4_IF/1

== system EB_12B_with_contracts/EB_12B_EBSpec/abs_call1111111111111111 ==
  abs_x : Inport  OutDataTypeStr=double
  branch_4_IF : Switch  Criteria=u2 ~= 0
  xxabs_1_operator : RelationalOperator  OutDataTypeStr=boolean  RndMeth=Simplest
  xxabs_1_rhs_2 : Constant  Value=0.0  OutDataTypeStr=double
  xxabs_2_operator : Gain  Gain=-1  OutDataTypeStr=double
  abs_y : Outport
  wires:
  branch_4_IF/1 -> abs_y/1
  xxabs_1_rhs_2/1 -> xxabs_1_operator/2
  xxabs_2_operator/1 -> branch_4_IF/3
  xxabs_1_operator/1 -> branch_4_IF/2
  abs_x/1 -> xxabs_2_operator/1, xxabs_1_operator/1, branch_4_IF/1

== system EB_12B_with_contracts/EB_12B_EBSpec/abs_call11111111111111111 ==
  abs_x : Inport  OutDataTypeStr=double
  branch_4_IF : Switch  Criteria=u2 ~= 0
  xxabs_1_operator : RelationalOperator  OutDataTypeStr=boolean  RndMeth=Simplest
  xxabs_1_rhs_2 : Constant  Value=0.0  OutDataTypeStr=double
  xxabs_2_operator : Gain  Gain=-1  OutDataTypeStr=double
  abs_y : Outport
  wires:
  branch_4_IF/1 -> abs_y/1
  xxabs_1_rhs_2/1 -> xxabs_1_operator/2
  xxabs_2_operator/1 -> branch_4_IF/3
  xxabs_1_operator/1 -> branch_4_IF/2
  abs_x/1 -> xxabs_2_operator/1, xxabs_1_operator/1, branch_4_IF/1

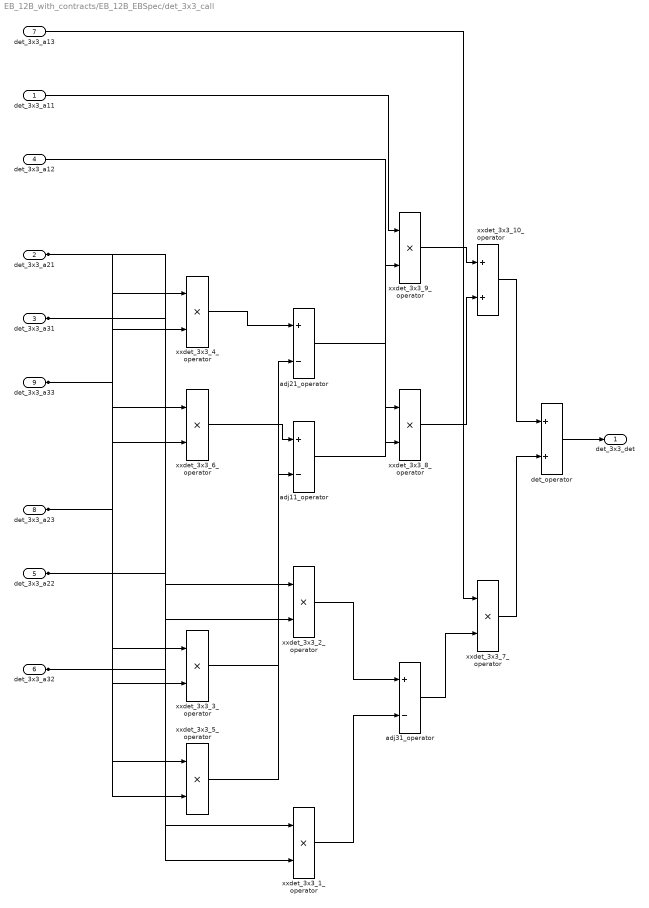
== system EB_12B_with_contracts/EB_12B_EBSpec/det_3x3_call ==
  det_3x3_a11 : Inport  OutDataTypeStr=double
  det_3x3_a21 : Inport  Port=2  OutDataTypeStr=double
  det_3x3_a31 : Inport  Port=3  OutDataTypeStr=double
  det_3x3_a12 : Inport  Port=4  OutDataTypeStr=double
  det_3x3_a22 : Inport  Port=5  OutDataTypeStr=double
  det_3x3_a32 : Inport  Port=6  OutDataTypeStr=double
  det_3x3_a13 : Inport  Port=7  OutDataTypeStr=double
  det_3x3_a23 : Inport  Port=8  OutDataTypeStr=double
  det_3x3_a33 : Inport  Port=9  OutDataTypeStr=double
  adj11_operator : Sum  Inputs=+-  OutDataTypeStr=double
  adj21_operator : Sum  Inputs=+-  OutDataTypeStr=double
  adj31_operator : Sum  Inputs=+-  OutDataTypeStr=double
  det_operator : Sum  OutDataTypeStr=double
  xxdet_3x3_10_operator : Sum  OutDataTypeStr=double
  xxdet_3x3_1_operator : Product  OutDataTypeStr=double
  xxdet_3x3_2_operator : Product  OutDataTypeStr=double
  xxdet_3x3_3_operator : Product  OutDataTypeStr=double
  xxdet_3x3_4_operator : Product  OutDataTypeStr=double
  xxdet_3x3_5_operator : Product  OutDataTypeStr=double
  xxdet_3x3_6_operator : Product  OutDataTypeStr=double
  xxdet_3x3_7_operator : Product  OutDataTypeStr=double
  xxdet_3x3_8_operator : Product  OutDataTypeStr=double
  xxdet_3x3_9_operator : Product  OutDataTypeStr=double
  det_3x3_det : Outport
  wires:
  det_operator/1 -> det_3x3_det/1
  adj11_operator/1 -> xxdet_3x3_9_operator/2
  det_3x3_a11/1 -> xxdet_3x3_9_operator/1
  adj21_operator/1 -> xxdet_3x3_8_operator/2
  det_3x3_a12/1 -> xxdet_3x3_8_operator/1
  adj31_operator/1 -> xxdet_3x3_7_operator/2
  det_3x3_a13/1 -> xxdet_3x3_7_operator/1
  xxdet_3x3_8_operator/1 -> xxdet_3x3_10_operator/2
  xxdet_3x3_9_operator/1 -> xxdet_3x3_10_operator/1
  xxdet_3x3_7_operator/1 -> det_operator/2
  xxdet_3x3_10_operator/1 -> det_operator/1
  xxdet_3x3_1_operator/1 -> adj31_operator/2
  xxdet_3x3_2_operator/1 -> adj31_operator/1
  xxdet_3x3_3_operator/1 -> adj21_operator/2
  xxdet_3x3_4_operator/1 -> adj21_operator/1
  xxdet_3x3_5_operator/1 -> adj11_operator/2
  xxdet_3x3_6_operator/1 -> adj11_operator/1
  det_3x3_a21/1 -> xxdet_3x3_3_operator/1, xxdet_3x3_2_operator/1
  det_3x3_a32/1 -> xxdet_3x3_5_operator/2, xxdet_3x3_2_operator/2
  det_3x3_a31/1 -> xxdet_3x3_4_operator/2, xxdet_3x3_1_operator/1
  det_3x3_a22/1 -> xxdet_3x3_6_operator/1, xxdet_3x3_1_operator/2
  det_3x3_a23/1 -> xxdet_3x3_5_operator/1, xxdet_3x3_4_operator/1
  det_3x3_a33/1 -> xxdet_3x3_6_operator/2, xxdet_3x3_3_operator/2

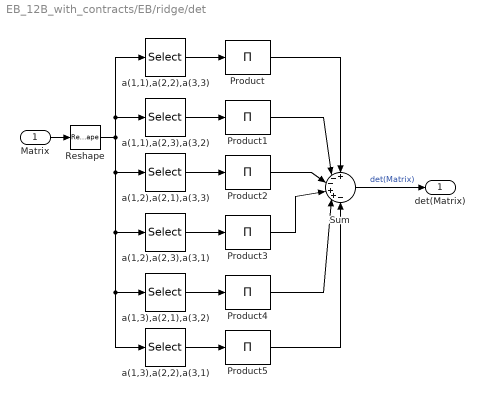
== system EB_12B_with_contracts/EB/ridge/det ==
  Matrix : Inport  PortDimensions=[3 3]
  Product{,1..5} (6 alike) : Product  Inputs=1  SaturateOnIntegerOverflow=on  OutDataTypeStr=Inherit: Same as first input
  Reshape : Reshape  OutputDimensionality=Column vector (2-D)
  Sum : Sum  Inputs=+--++-  SaturateOnIntegerOverflow=on
  a(1,1),a(2,2),a(3,3) : Selector  InputPortWidth=9  IndexOptions=Index vector (dialog)  Indices=[1 5 9]  OutputSizes=1
  a(1,1),a(2,3),a(3,2) : Selector  InputPortWidth=9  IndexOptions=Index vector (dialog)  Indices=[1 6 8]  OutputSizes=1
  a(1,2),a(2,1),a(3,3) : Selector  InputPortWidth=9  IndexOptions=Index vector (dialog)  Indices=[2 4 9]  OutputSizes=1
  a(1,2),a(2,3),a(3,1) : Selector  InputPortWidth=9  IndexOptions=Index vector (dialog)  Indices=[3 4 8]  OutputSizes=1
  a(1,3),a(2,1),a(3,2) : Selector  InputPortWidth=9  IndexOptions=Index vector (dialog)  Indices=[2 6 7]  OutputSizes=1
  a(1,3),a(2,2),a(3,1) : Selector  InputPortWidth=9  IndexOptions=Index vector (dialog)  Indices=[3 5 7]  OutputSizes=1
  det(Matrix) : Outport  PortDimensions=1  VectorParamsAs1DForOutWhenUnconnected=off
  wires:
  a(1,1),a(2,2),a(3,3)/1 -> Product/1
  a(1,1),a(2,3),a(3,2)/1 -> Product1/1
  a(1,2),a(2,1),a(3,3)/1 -> Product2/1
  a(1,2),a(2,3),a(3,1)/1 -> Product3/1
  a(1,3),a(2,1),a(3,2)/1 -> Product4/1
  a(1,3),a(2,2),a(3,1)/1 -> Product5/1
  Product/1 -> Sum/1
  Product1/1 -> Sum/2
  Product2/1 -> Sum/3
  Product3/1 -> Sum/4
  Product4/1 -> Sum/5
  Product5/1 -> Sum/6
  Matrix/1 -> Reshape/1
  Sum/1 -> det(Matrix)/1  "det(Matrix)"
  Reshape/1 -> a(1,1),a(2,2),a(3,3)/1, a(1,1),a(2,3),a(3,2)/1, a(1,2),a(2,1),a(3,3)/1, a(1,2),a(2,3),a(3,1)/1, a(1,3),a(2,1),a(3,2)/1, a(1,3),a(2,2),a(3,1)/1
